simulink model "localization"  (R2019b)
settings: Solver=FixedStepAuto  StartTime=0.0  StopTime=310  FixedStep=sample_time  RelTol=1e-3
PreLoadFcn:
  | initLocalization
InitFcn:
  | initLocalization
  | insertArtificialOutages
StopFcn:
  | simout_data_prepared = false;
  | map_data_prepared = false;
  | % prepareSimOutData
undefined symbols (not defined in the file or in its folder): a_bias_gain, a_e_limit, a_e_ma_time, d_bogies, E_w_limit, E_w_ma_time, gnss_lever_arm, gnss_sample_time, gnss_speed_limit, imm_sample_time, p_llh_n_0_rad, psi_0, Q_arc, q_b_n_0, Q_imm, Q_imm_trash, Q_straight, sample_time, sigma_v_acc, sigma_v_gyro, v_min_tgc, v_ned_eb_n_0, w_bias_gain
libraries: libMdl_RecordedData x4, libMdl_quatToEuler x3, simulink x2, libMdl_InsBiasEstimator x2, libMdl_Imm x1, libMdl_KalmanFilter x1, libMdl_invQuat x1, libMdl_GnssDataCorrector x1, libMdl_ImuDataCorrector x1, libMdl_AccIntegrator x1, libMdl_AttitudeComputer x1, libMdl_CarriageMisalignment x1
(part 2 of 2)

== matlab function localization/Localization Filter/Parameter Identification, Localization Correction and Map Building/Map Building/Railway Map Builder ==
  data: geometry input; topology output size=[max_track_map_size max_track_map_size]; reset_flag input; s input; P_s input; l_old input; track_start_points output size=[max_track_map_size 5]; P_track_start_points output size=[3 3 max_track_map_size]; track_maps output size=[max_track_map_size 7]; P_track_maps output size=[3 3 max_track_map_size]; optimization_data_selector output size=[max_track_map_size 2]; max_track_map_size parameter
function [topology,track_start_points,P_track_start_points,track_maps,P_track_maps,optimization_data_selector] = simFcn_BuildRaiwlayMap(geometry,reset_flag,s,P_s,l_old,max_track_map_size)

% % Init ____________________________________________________________________
% 
% coder.extrinsic('simFcn_TgcMapBuilding');
% 
% coder.varsize('topology',[max_track_map_size max_track_map_size]);
% coder.varsize('track_start_points',[max_track_map_size 5]);
% coder.varsize('P_track_start_points',[3 3 max_track_map_size]);
% coder.varsize('track_maps',[max_track_map_size 7]);
% coder.varsize('P_track_maps',[3 3 max_track_map_size]);
% coder.varsize('optimization_data_selector',[max_track_map_size 2]);
% 
% % Calculations ____________________________________________________________
% 
% [topology_from_fcn,track_start_points_from_fcn,P_track_start_points_from_fcn,track_maps_from_fcn,P_track_maps_from_fcn,optimization_data_selector_from_fcn] = simFcn_TgcMapBuilding(geometry,reset_flag,s,P_s,max_track_map_size);
% 
% % See:
% % https://stackoverflow.com/questions/29721819/problems-with-using-mxarrays-with-the-step-function-in-matlab-coder/29725862?iemail=1&noredirect=1#29725862
% dims_topology_estm = zeros(1,2);
% dims_topology_estm = size(topology_from_fcn);
% topology = coder.nullcopy(zeros(dims_topology_estm));
% topology = topology_from_fcn;
% 
% dims_track_start_points = zeros(1,2);
% dims_track_start_points = size(track_start_points_from_fcn);
% track_start_points = coder.nullcopy(zeros(dims_track_start_points));
% track_start_points = track_start_points_from_fcn;
% 
% dims_P_track_start_points = zeros(1,3);
% dims_P_track_start_points = [size(P_track_start_points_from_fcn,1), size(P_track_start_points_from_fcn,2), size(P_track_start_points_from_fcn,3)];
% P_track_start_points = coder.nullcopy(zeros(dims_P_track_start_points));
% P_track_start_points = P_track_start_points_from_fcn;
% 
% dims_track_map = zeros(1,2);
% dims_track_map = size(track_maps_from_fcn);
% track_maps = coder.nullcopy(zeros(dims_track_map));
% track_maps = track_maps_from_fcn;
% 
% dims_P_track_map = zeros(1,3);
% dims_P_track_map = [size(P_track_maps_from_fcn,1), size(P_track_maps_from_fcn,2), size(P_track_maps_from_fcn,3)];
% P_track_maps = coder.nullcopy(zeros(dims_P_track_map));
% P_track_maps = P_track_maps_from_fcn;
% 
% dims_optimization_data_selector = zeros(1,2);
% dims_optimization_data_selector = size(optimization_data_selector_from_fcn);
% optimization_data_selector = coder.nullcopy(zeros(dims_optimization_data_selector));
% optimization_data_selector = optimization_data_selector_from_fcn;

coder.varsize('mem_var_topology',[max_track_map_size max_track_map_size]);
coder.varsize('mem_var_track_start_points',[max_track_map_size 5]);
coder.varsize('mem_var_P_track_start_points',[3 3 max_track_map_size]);
coder.varsize('mem_var_track_maps',[max_track_map_size 7]);
coder.varsize('mem_var_P_track_maps',[3 3 max_track_map_size]);
coder.varsize('mem_var_optimization_data_selector',[max_track_map_size 2]);

%% Initialization and checks

% persistent mem_var_railway_map
persistent mem_var_topology mem_var_track_start_points mem_var_P_track_start_points mem_var_track_maps mem_var_P_track_maps
persistent mem_var_map_optimization_data_index
persistent mem_var_optimization_data_selector 
persistent mem_var_unkown_track_dir_corrected

empty_track_start_point = @(id) [id nan nan nan];
empty_P_track_start_point = nan(3);
empty_track_map = @(id) [id nan nan nan nan nan];
empty_P_track_map = nan(3);

% Initialize railway-map on first run _____________________________________
if isempty(mem_var_topology)    
       
    initial_track_id = 1;
    mem_var_topology = 0;
    mem_var_track_start_points = empty_track_start_point(initial_track_id);
    mem_var_P_track_start_points = cat(3,empty_P_track_start_point);
    mem_var_track_maps = empty_track_map(initial_track_id);
    mem_var_P_track_maps = cat(3,empty_P_track_map);
        
    current_track_id = initial_track_id;

% Extend railway-map if necessary _________________________________________
else    
    
    current_track_id = mem_var_track_start_points(end,1);
    current_map_size = length(mem_var_topology);
    
    % 1) append current trackmap with know track __________________________
    if reset_flag 
        
%         test_idx = max(size(mem_var_track_maps,1)-1,1);
%         if isnan(mem_var_track_maps(end,2)) && isnan(mem_var_track_maps(test_idx,2))
%             test = 1;
%         end % if
        
        % Uptate track-length of old track
        mem_var_track_maps(end,5) = abs(l_old(1));
        mem_var_P_track_maps(3,3,end) = l_old(2); 
        
        % Append
        current_track_id = current_track_id + 1;        
        mem_var_topology = [zeros(current_map_size,1) eye(current_map_size); zeros(1,current_map_size+1)];
        mem_var_track_start_points = [mem_var_track_start_points; empty_track_start_point(current_track_id)];
        mem_var_P_track_start_points = cat(3,mem_var_P_track_start_points,empty_P_track_start_point);
        mem_var_track_maps = [mem_var_track_maps; empty_track_map(current_track_id)];
        mem_var_P_track_maps = cat(3,mem_var_P_track_maps,empty_P_track_map);
                
    end % if    
    
end % if

% Initialize map optimization variables ___________________________________
if isempty(mem_var_map_optimization_data_index)
    mem_var_map_optimization_data_index = 1;    
else
    mem_var_map_optimization_data_index = max(mem_var_map_optimization_data_index + 1,1);
end % if

if isempty(mem_var_optimization_data_selector)
    mem_var_optimization_data_selector = zeros(1,2);
end % if

% Initialize other variables ______________________________________________

if isempty(mem_var_unkown_track_dir_corrected)
    mem_var_unkown_track_dir_corrected = false;
end % if

%% Calculations

% Fill Railway-Map ________________________________________________________
switch geometry
    
    case 1 % straight _____________________________________________________
               
        % Start point
        mem_var_track_start_points(end,2) = s(3);
        mem_var_track_start_points(end,3) = s(4);
        mem_var_track_start_points(end,4) = rad2deg(pi/2-s(5)); % Transformation needed to meet Railway Toolbox implementation
        mem_var_P_track_start_points(:,:,end) = blkdiag(P_s(3:4,3:4),rad2deg(P_s(5,5)));
        
        % Trackmap        
        mem_var_track_maps(end,2) = geometry;
        mem_var_track_maps(end,3) = 0;
        mem_var_track_maps(end,4) = 0;
        mem_var_track_maps(end,5) = abs(s(7));
        mem_var_track_maps(end,6) = calcSpeedLimit(160,0);
        mem_var_P_track_maps(:,:,end) = diag([0 0 P_s(7,7)]); 
                    
    case 3 % circular arc _________________________________________________
        
        % Start point
        mem_var_track_start_points(end,2) = s(3);
        mem_var_track_start_points(end,3) = s(4);
        mem_var_track_start_points(end,4) = rad2deg(pi/2-s(5)); % Transformation needed to meet Railway Toolbox implementation
        mem_var_P_track_start_points(:,:,end) = blkdiag(P_s(3:4,3:4),P_s(7,7));

        % Trackmap       
        mem_var_track_maps(end,2) = geometry;
        mem_var_track_maps(end,3) = s(6);
        mem_var_track_maps(end,4) = s(6);
        mem_var_track_maps(end,5) = abs(s(7));
        mem_var_track_maps(end,6) =  calcSpeedLimit(160,s(6));
        mem_var_P_track_maps(:,:,end) = diag([0 P_s(6,6) P_s(7,7)]);
           
    otherwise % undefined geometry ________________________________________
                
        if reset_flag || any(isnan(mem_var_track_start_points(end,:)))                
            mem_var_track_start_points(end,2) = s(3);
            mem_var_track_start_points(end,3) = s(4);
            mem_var_track_start_points(end,4) = rad2deg(pi/2-s(5)); % Transformation needed to meet Railway Toolbox implementation
            mem_var_P_track_start_points(:,:,end) = blkdiag(P_s(3:4,3:4),P_s(7,7));
        end % if        
                
        mem_var_track_maps(end,5) = abs(s(7));
        mem_var_P_track_maps(:,:,end) = diag([0 0 P_s(7,7)]);
        
end % switch

% Consider reverse driving ________________________________________________

if s(7) < 0
    
    if isnan(mem_var_track_maps(end,2)) && ~mem_var_unkown_track_dir_corrected
        mem_var_track_start_points(end,4) = mem_var_track_start_points(end,4)-180;
        mem_var_unkown_track_dir_corrected = true;
    elseif ~isnan(mem_var_track_maps(end,2)) 
        mem_var_track_start_points(end,4) = mem_var_track_start_points(end,4)-180;
        mem_var_unkown_track_dir_corrected = false;
    end % if        

    mem_var_track_maps(end,3) = -mem_var_track_maps(end,3);
    mem_var_track_maps(end,4) = -mem_var_track_maps(end,4);
end % if

% Prepare later map optimization __________________________________________
track_map_index = size(mem_var_track_maps,1);
if track_map_index > size(mem_var_optimization_data_selector,1)
    mem_var_optimization_data_selector = [mem_var_optimization_data_selector; current_track_id mem_var_map_optimization_data_index];
else
    mem_var_optimization_data_selector(track_map_index,:) = [current_track_id mem_var_map_optimization_data_index];
end % if

%% Output

topology = mem_var_topology;
track_start_points = mem_var_track_start_points;
P_track_start_points = mem_var_P_track_start_points;
track_maps = mem_var_track_maps;
P_track_maps = mem_var_P_track_maps;
optimization_data_selector = mem_var_optimization_data_selector;

%% Final checks

if length(unique(mem_var_track_start_points(:,1))) ~= length(mem_var_track_start_points(:,1))
    error('simFcn_GeomParamEstimation: Error in track-start-points, the IDs have to be unique!');
end %if

end % function

== matlab function localization/Localization Filter/Parameter Identification, Localization Correction and Map Building/Correction Data Preparation/Data Preparation ==
  data: enable input; x_imm input; geometry output; P_imm input; mu input; z input; R input; reset_flag output; s_0 output; P_s_0 output; z_s output; R_s output; l_old output; d_bogies input; gamma output; v_min_tgc input
function [geometry,reset_flag,s_0,P_s_0,z_s,R_s,l_old,gamma] = simFcn_DataPreparation(enable,x_imm,P_imm,mu,z,R,d_bogies,v_min_tgc)

% Init ____________________________________________________________________

% coder.extrinsic('simFcn_TgcDataPreparation');

geometry = coder.nullcopy(zeros(1,1));
reset_flag = coder.nullcopy(zeros(1,1));
s_0 = coder.nullcopy(zeros(8,1));
P_s_0 = coder.nullcopy(zeros(8,8));
z_s = coder.nullcopy(zeros(4,1));
R_s = coder.nullcopy(zeros(4,4));
l_old = coder.nullcopy(zeros(2,1));
gamma = coder.nullcopy(zeros(1,1));

% Calculations ____________________________________________________________

[geometry,reset_flag,s_0,P_s_0,z_s,R_s,l_old,gamma] = simFcn_TgcDataPreparation(enable,x_imm,P_imm,mu,z,R,d_bogies,v_min_tgc);

end % function

== matlab function localization/Strapdown Calculations/Strapdown Calculations/Quaternion Integration/simQuaternionIntegration ==
  data: q_b_n_prev input; w_nb_b input; standstill_flag input size=1; q_b_n output; T input
function q_b_n = fcn(q_b_n_prev,w_nb_b,standstill_flag,T)
% See:  D. Titterton and J. Westen, "Strapdown Inertial Navigation Technology", pp. 319-320, IET, 2004
%

if 0 == standstill_flag
    
    sigma = w_nb_b.*T;
    sigma_norm = sqrt(sum(sigma.^2));

    a_c = cos(sigma_norm/2);
    if sigma_norm > 1e-3
        a_s = sin(sigma_norm/2)/sigma_norm;
    else
        a_s = 0.5;
    end % if

    q_k = q_b_n_prev;
    r_k = [a_c;a_s.*sigma];
    q_k_new = multQuat(q_k,r_k);

    q_b_n = normalizeQuat(q_k_new);

else
   
    q_b_n = q_b_n_prev;
    
end % if

end % function
